simulink model "motor2"  (R2022b)
settings: Solver=ode45  StartTime=0.0  StopTime=3  MaxStep=0.0001  RelTol=1e-3
undefined symbols (not defined in the file or in its folder): awu, dac, degs2rpm, diff, ff, in, National_Instruments, PCIe, pid, rpm2rads, sens
libraries: sldrtlib x3, simulink x1
settings Model: Creator=loren  LastModifiedBy=loren
settings DataIOCC: ReturnWorkspaceOutputs=off
settings ModelReferenceCC: EnableRefExpFcnMdlSchedulingChecks=on

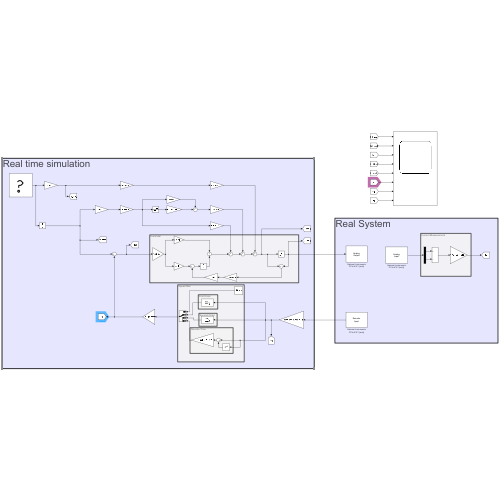
[thumbnail: Simulink's stored preview of the top-level diagram]
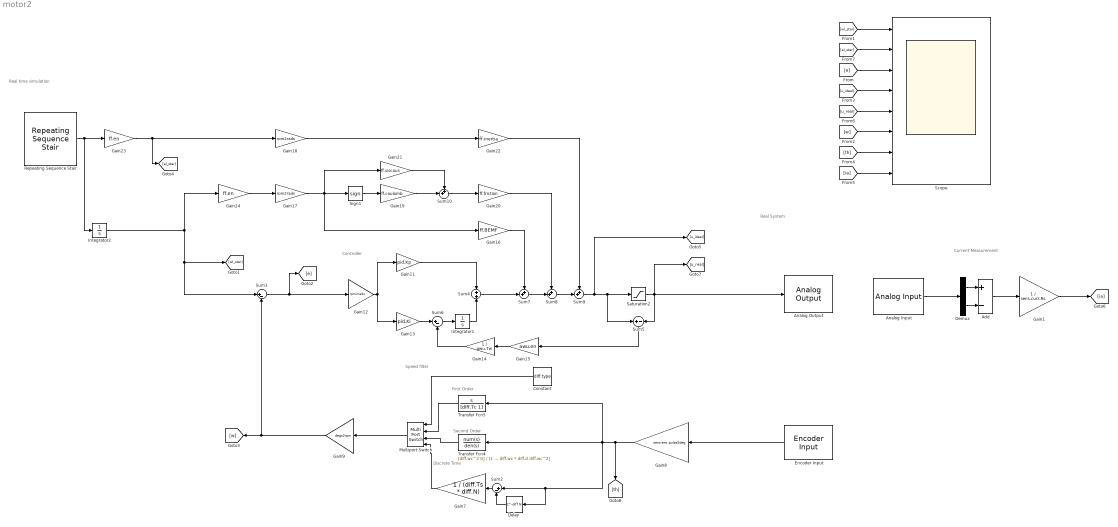
== system motor2 ==
  note: Real time simulation
  note: Controller
  note: Speed filter
  note: Discrete Time
  note: Second Order
  note: First Order
  note: Current Measurement
  note: Real System
  Add : Sum  Inputs=+-
  Analog Input : sldrtlib/Analog Input  SampleTime=-1  MaxMissedTicks=10  ShowMissedTicks=off  YieldWhenWaiting=off  DrvName=National_Instruments/PCIe-6321  DrvAddress=4294967295  DrvOptions=[0 0 0 2 0 0 0]  Channels=[1 2]  RangeMode=1  VoltRange=1  DataType=1
      settings: AttributesFormatString=National Instruments\nPCIe-6321 [auto]
  Analog Output : sldrtlib/Analog Output  SampleTime=-1  MaxMissedTicks=10  ShowMissedTicks=off  YieldWhenWaiting=off  DrvName=National_Instruments/PCIe-6321  DrvAddress=4294967295  DrvOptions=[0 0 0 2 0 0 0]  Channels=1  RangeMode=1  VoltRange=1  InitialValue=0  FinalValue=0
      settings: AttributesFormatString=National Instruments\nPCIe-6321 [auto]
  Constant : Constant  Value=diff.type
  Delay : Delay  DelayLength=diff.N
  Demux : Demux  Outputs=2
  Encoder Input : sldrtlib/Encoder Input  SampleTime=-1  MaxMissedTicks=10  ShowMissedTicks=off  YieldWhenWaiting=off  DrvName=National_Instruments/PCIe-6321  DrvAddress=4294967295  DrvOptions=[0 0 0 2 0 0 0]  Channels=1  QuadMode=3  IndexPulse=1  InputFilter=Inf  DataType=1
      settings: AttributesFormatString=National Instruments\nPCIe-6321 [auto]
  Gain1 : Gain  Gain=1 / sens.curr.Rs
  Gain11 : Gain  Gain=pid.Kp
  Gain12 : Gain  Gain=rpm2rads
  Gain13 : Gain  Gain=pid.Ki
  Gain14 : Gain  Gain=1 / awu.Tw
  Gain15 : Gain  Gain=awu.en
  Gain16 : Gain  Gain=ff.BEMF
  Gain17 : Gain  Gain=rpm2rads
  Gain18 : Gain  Gain=rpm2rads
  Gain19 : Gain  Gain=ff.coulomb
  Gain20 : Gain  Gain=ff.friction
  Gain21 : Gain  Gain=ff.viscous
  Gain22 : Gain  Gain=ff.inertia
  Gain23 : Gain  Gain=ff.en
  Gain24 : Gain  Gain=ff.en
  Gain7 : Gain  Gain=1 / (diff.Ts * diff.N)
  Gain8 : Gain  Gain=sens.enc.pulse2deg
  Gain9 : Gain  Gain=degs2rpm
  Integrator1 : Integrator
  Integrator2 : Integrator
  Multiport Switch : MultiPortSwitch  SaturateOnIntegerOverflow=off  InputSameDT=off
  Repeating Sequence Stair : simulink/Sources/Repeating Sequence Stair  OutValues=[in.a 0 -in.a -in.a 0 in.a].'  tsamp=in.t  OutMin=[]  OutMax=[]  OutDataTypeStr=double  OutputDataTypeScalingMode=double  OutDataType=fixdt(0,8)  ConRadixGroup=Best Precision: Vector-wise  OutScaling=2^-12
  Saturation2 : Saturate  UpperLimit=dac.V  LowerLimit=-dac.V
  Scope : Scope  NumInputPorts=8
  Sign1 : Signum  ZeroCross=off
  Sum{7..10} (4 alike) : Sum  Inputs=++|
  Sum2 : Sum  Inputs=|+-
  Sum3 : Sum  Inputs=|+-
  Sum4 : Sum  Inputs=+|+
  Sum5 : Sum  Inputs=+|-
  Sum6 : Sum  Inputs=|+-
  Transfer Fcn4 : TransferFcn  Numerator=[diff.wc^2 0]  Denominator=[1 2 * diff.wc * diff.d diff.wc^2]
  Transfer Fcn5 : TransferFcn  Numerator=[1 0]  Denominator=[diff.Tc 1]
  wires:
  Gain8/1 -> Delay/1, Sum2/1, Transfer Fcn4/1, Transfer Fcn5/1, [th]
  Delay/1 -> Sum2/2
  Sum2/1 -> Gain7/1
  Multiport Switch/1 -> Gain9/1
  Transfer Fcn5/1 -> Multiport Switch/2
  Transfer Fcn4/1 -> Multiport Switch/3
  Constant/1 -> Multiport Switch/1
  Gain9/1 -> [w], Sum3/2
  Sum3/1 -> [e], Gain12/1
  Gain12/1 -> Gain11/1, Gain13/1
  Gain11/1 -> Sum4/1
  Integrator1/1 -> Sum4/2
  Gain7/1 -> Multiport Switch/4
  Integrator2/1 -> [wl_star], Sum3/1, Gain24/1
  Gain13/1 -> Sum6/1
  Sum6/1 -> Integrator1/1
  Saturation2/1 -> [u_real], Analog Output/1, Sum5/2
  Sum5/1 -> Gain15/1
  Gain14/1 -> Sum6/2
  Gain15/1 -> Gain14/1
  Sum8/1 -> Sum9/2
  Sum7/1 -> Sum8/2
  Sum4/1 -> Sum7/2
  Sum9/1 -> [u_ideal], Sum5/1, Saturation2/1
  Gain16/1 -> Sum7/1
  Gain20/1 -> Sum8/1
  Gain22/1 -> Sum9/1
  Sum10/1 -> Gain20/1
  Gain21/1 -> Sum10/1
  Gain19/1 -> Sum10/2
  Sign1/1 -> Gain19/1
  Gain17/1 -> Gain16/1, Gain21/1, Sign1/1
  Gain18/1 -> Gain22/1
  Repeating Sequence Stair/1 -> Gain23/1, Integrator2/1
  Gain23/1 -> [al_star], Gain18/1
  Gain24/1 -> Gain17/1
  Demux/1 -> Add/1
  Analog Input/1 -> Demux/1
  Gain1/1 -> [ia]
  Add/1 -> Gain1/1
  Demux/2 -> Add/2
  Encoder Input/1 -> Gain8/1
  [e] -> Scope/3
  [w] -> Scope/6
  [u_ideal] -> Scope/4
  [u_real] -> Scope/5
  [wl_star] -> Scope/1
  [th] -> Scope/7
  [ia] -> Scope/8
  [al_star] -> Scope/2
